simulink model "rotor_simulink"  (R2022a)
settings: Solver=VariableStepAuto  StartTime=0.1  StopTime=60  FixedStep=sample_time/10  RelTol=1e-3
values from neighbouring files (symbols this model uses):
  B_eq = rotor.B + generator.B/gearbox.ratio^2    [parameters.m]
  I_eq = rotor.I/gearbox.ratio^2 + generator.I    [main.m]    (also in parameters.m = rotor.I + generator.I/gearbox.ratio^2)
  lambda_opt = lambda_vector(lambda_pos)    [lookup_cp.m]    (also in mesh_cp.m; parameters.m = rated_values(4); reference_selection.m = 7.857)
  lambda_vector = linspace(lambda_range(1), lambda_range(2), lambda_item)    [mesh_cp.m]    (also in parameters.m)
  lookup_Pitch = zeros(3, velocity_item)    [lookup_pitch.m]    (also in lookup_pitch.mat = [0 0 0 0.5 0 0 1 0 0 1.5 0 0 ... (183 elements, 3x61)])
  omega_rated = V0_rated*lambda_opt/rotor.R    [lookup_cp.m]    (also in mesh_cp.m; parameters.m = rated_values(2); reference_selection.m = 1.008234212)
  pitch_vector = linspace(pitch_range(1), pitch_range(2), pitch_item)    [mesh_cp.m]    (also in parameters.m)
  rated_values = [11.4382324778 1.03294686619 9.86391598231 8.05263157895 0.46469860786]    [rated_values.mat]
  rho = 1.225    [main.m]    (also in parameters.m; reference_selection.m)
  sample_time = wind_speed(2,1) - wind_speed(1, 1)    [main.m]    (also in parameters.m)
  V0_rated = (rotor.P_rated/(0.5*rho*cP_max*rotor.A))^(1/3)    [lookup_cp.m]    (also in mesh_cp.m; parameters.m = rated_values(1); reference_selection.m = 11.44)
  velocity_vector = sort(velocity_vector)    [parameters.m]
  wind_speed = load('usim.dat')    [main.m]    (also in parameters.m; rotor_test.m = 25)
undefined symbols (not defined in the file or in its folder): blade, gearbox, generator, lookup_cP, omega_r, rotor
settings Model: Creator=Niccolò  LastModifiedBy=Niccolò

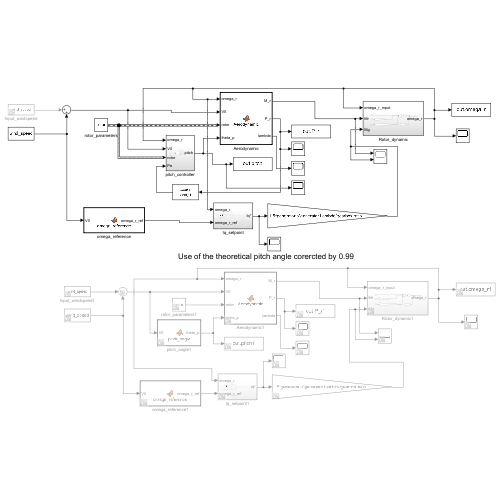
[thumbnail: Simulink's stored preview of the top-level diagram]
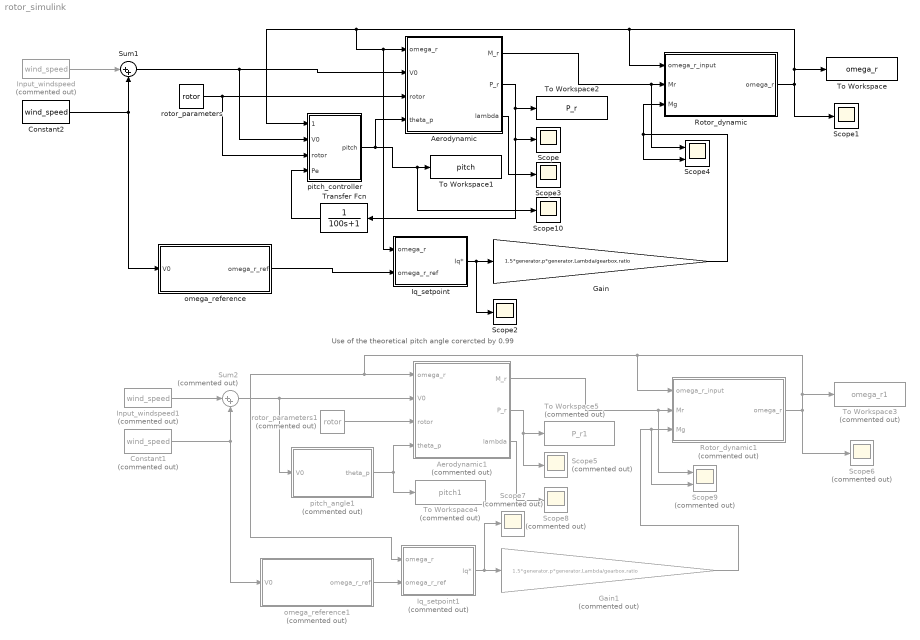
== system rotor_simulink ==
  note: Use of the theoretical pitch angle corercted by 0.99
  Aerodynamic : MATLAB Function  TreatAsAtomicUnit=on
  Aerodynamic1 : MATLAB Function  Commented=on  TreatAsAtomicUnit=on
  Constant1 : Constant  Commented=on  Value=wind_speed
  Constant2 : Constant  Value=wind_speed
  Gain : Gain  Gain=1.5*generator.p*generator.Lambda/gearbox.ratio
  Gain1 : Gain  Commented=on  Gain=1.5*generator.p*generator.Lambda/gearbox.ratio
  Input_windspeed : FromWorkspace  Commented=on  VariableName=wind_speed  SampleTime=sample_time
  Input_windspeed1 : FromWorkspace  Commented=on  VariableName=wind_speed  SampleTime=sample_time
  Iq_setpoint : Subsystem
  Iq_setpoint1 : Subsystem  Commented=on
  Rotor_dynamic : Subsystem
  Rotor_dynamic1 : Subsystem  Commented=on
  Scope{,1..3,10} (5 alike) : Scope
  Scope4 : Scope  NumInputPorts=2
  Scope{5..8} (4 alike) : Scope  Commented=on
  Scope9 : Scope  Commented=on  NumInputPorts=2
  Sum1 : Sum  Inputs=|++
  Sum2 : Sum  Commented=on  Inputs=|++
  To Workspace : ToWorkspace  VariableName=omega_r  SaveFormat=Timeseries  SampleTime=-1
  To Workspace1 : ToWorkspace  VariableName=pitch  SaveFormat=Timeseries  SampleTime=-1
  To Workspace2 : ToWorkspace  VariableName=P_r  SaveFormat=Timeseries  SampleTime=-1
  To Workspace3 : ToWorkspace  Commented=on  VariableName=omega_r1  SaveFormat=Timeseries  SampleTime=-1
  To Workspace4 : ToWorkspace  Commented=on  VariableName=pitch1  SaveFormat=Timeseries  SampleTime=-1
  To Workspace5 : ToWorkspace  Commented=on  VariableName=P_r1  SaveFormat=Timeseries  SampleTime=-1
  Transfer Fcn : TransferFcn  Denominator=[100 1]
  omega_reference : MATLAB Function  TreatAsAtomicUnit=on
  omega_reference1 : MATLAB Function  Commented=on  TreatAsAtomicUnit=on
  pitch_angle1 : MATLAB Function  Commented=on  TreatAsAtomicUnit=on
  pitch_controller : Subsystem
  rotor_parameters : Constant  Value=rotor  OutDataTypeStr=Bus: rotor_bus
  rotor_parameters1 : Constant  Commented=on  Value=rotor  OutDataTypeStr=Bus: rotor_bus
  wires:
  Input_windspeed/1 -> Sum1/1
  rotor_parameters/1 -> pitch_controller/3(rotor), Aerodynamic/3(rotor)
  Constant2/1 -> omega_reference/1(V0), Sum1/2
  omega_reference/1(omega_r_ref) -> Iq_setpoint/2(omega_r_ref)
  Iq_setpoint/1(Iq*) -> Scope2/1, Gain/1
  Gain/1 -> Rotor_dynamic/3(Mg), Scope4/2
  Aerodynamic/1(M_r) -> Scope4/1, Rotor_dynamic/2(Mr)
  Sum1/1 -> Aerodynamic/2(V0), pitch_controller/2(V0)
  Aerodynamic/3(lambda) -> Scope3/1
  Aerodynamic1/3(lambda) -> Scope8/1
  Constant1/1 -> omega_reference1/1(V0), Sum2/2
  Input_windspeed1/1 -> Sum2/1
  Sum2/1 -> Aerodynamic1/2(V0), pitch_angle1/1(V0)
  rotor_parameters1/1 -> Aerodynamic1/3(rotor)
  pitch_angle1/1(theta_p) -> Aerodynamic1/4(theta_p), To Workspace4/1
  Rotor_dynamic1/1(omega_r) -> Rotor_dynamic1/1(omega_r_input), Iq_setpoint1/1(omega_r), Aerodynamic1/1(omega_r), To Workspace3/1, Scope6/1
  omega_reference1/1(omega_r_ref) -> Iq_setpoint1/2(omega_r_ref)
  Gain1/1 -> Scope9/2, Rotor_dynamic1/3(Mg)
  Iq_setpoint1/1(Iq*) -> Scope7/1, Gain1/1
  Aerodynamic1/2(P_r) -> Scope5/1, To Workspace5/1
  Aerodynamic1/1(M_r) -> Scope9/1, Rotor_dynamic1/2(Mr)
  Aerodynamic/2(P_r) -> Transfer Fcn/1, Scope/1, To Workspace2/1
  Rotor_dynamic/1(omega_r) -> Rotor_dynamic/1(omega_r_input), pitch_controller/1(omega_r), Iq_setpoint/1(omega_r), Aerodynamic/1(omega_r), To Workspace/1, Scope1/1
  pitch_controller/1(pitch) -> Aerodynamic/4(theta_p), Scope10/1, To Workspace1/1
  Transfer Fcn/1 -> pitch_controller/4(Pe)

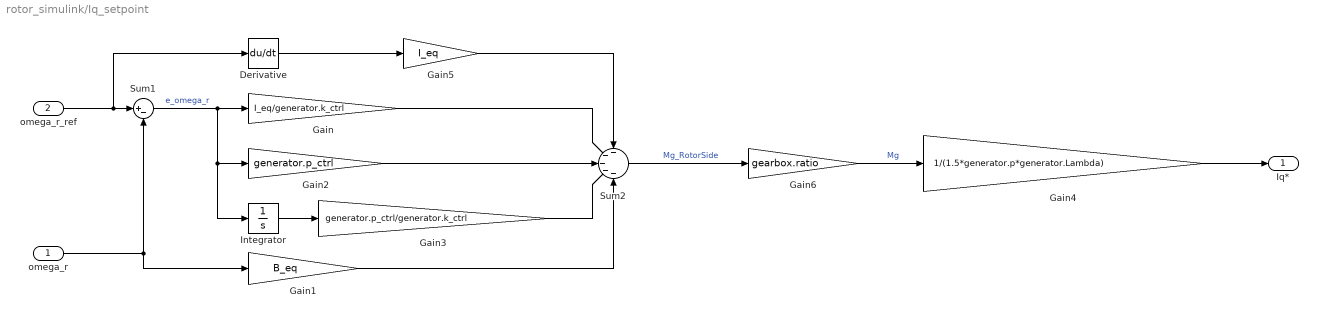
== system rotor_simulink/Iq_setpoint ==
  omega_r : Inport
  omega_r_ref : Inport  Port=2
  Derivative : Derivative
  Gain : Gain  Gain=I_eq/generator.k_ctrl
  Gain1 : Gain  Gain=B_eq
  Gain2 : Gain  Gain=generator.p_ctrl
  Gain3 : Gain  Gain=generator.p_ctrl/generator.k_ctrl
  Gain4 : Gain  Gain=1/(1.5*generator.p*generator.Lambda)
  Gain5 : Gain  Gain=I_eq
  Gain6 : Gain  Gain=gearbox.ratio
  Integrator : Integrator
  Sum1 : Sum  Inputs=|+-
  Sum2 : Sum  Inputs=-----
  Iq* : Outport
  wires:
  Gain/1 -> Sum2/2
  Sum1/1 -> Integrator/1, Gain2/1, Gain/1  "e_omega_r"
  Gain1/1 -> Sum2/5
  Gain4/1 -> Iq*/1
  omega_r_ref/1 -> Derivative/1, Sum1/1
  omega_r/1 -> Gain1/1, Sum1/2
  Integrator/1 -> Gain3/1
  Gain3/1 -> Sum2/4
  Gain2/1 -> Sum2/3
  Sum2/1 -> Gain6/1  "Mg_RotorSide"
  Gain5/1 -> Sum2/1
  Gain6/1 -> Gain4/1  "Mg"
  Derivative/1 -> Gain5/1

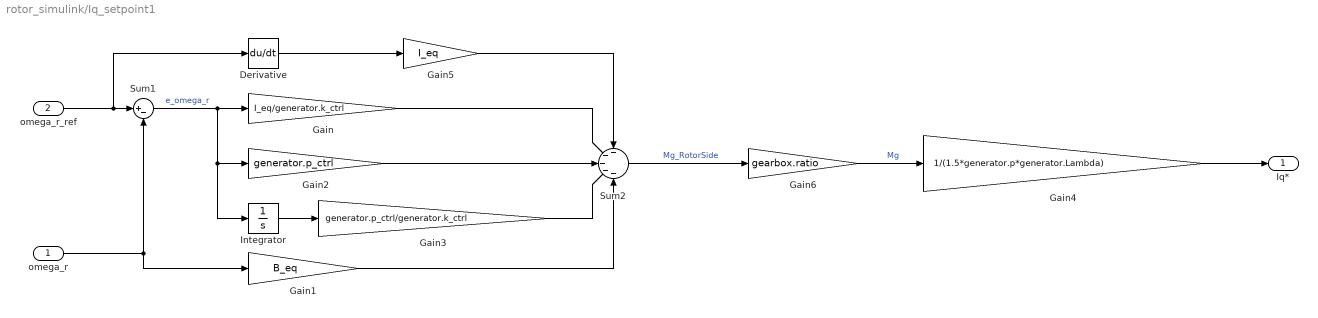
== system rotor_simulink/Iq_setpoint1 ==
  omega_r : Inport
  omega_r_ref : Inport  Port=2
  Derivative : Derivative
  Gain : Gain  Gain=I_eq/generator.k_ctrl
  Gain1 : Gain  Gain=B_eq
  Gain2 : Gain  Gain=generator.p_ctrl
  Gain3 : Gain  Gain=generator.p_ctrl/generator.k_ctrl
  Gain4 : Gain  Gain=1/(1.5*generator.p*generator.Lambda)
  Gain5 : Gain  Gain=I_eq
  Gain6 : Gain  Gain=gearbox.ratio
  Integrator : Integrator
  Sum1 : Sum  Inputs=|+-
  Sum2 : Sum  Inputs=-----
  Iq* : Outport
  wires:
  Gain/1 -> Sum2/2
  Sum1/1 -> Integrator/1, Gain2/1, Gain/1  "e_omega_r"
  Gain1/1 -> Sum2/5
  Gain4/1 -> Iq*/1
  omega_r_ref/1 -> Derivative/1, Sum1/1
  omega_r/1 -> Gain1/1, Sum1/2
  Integrator/1 -> Gain3/1
  Gain3/1 -> Sum2/4
  Gain2/1 -> Sum2/3
  Sum2/1 -> Gain6/1  "Mg_RotorSide"
  Gain5/1 -> Sum2/1
  Gain6/1 -> Gain4/1  "Mg"
  Derivative/1 -> Gain5/1

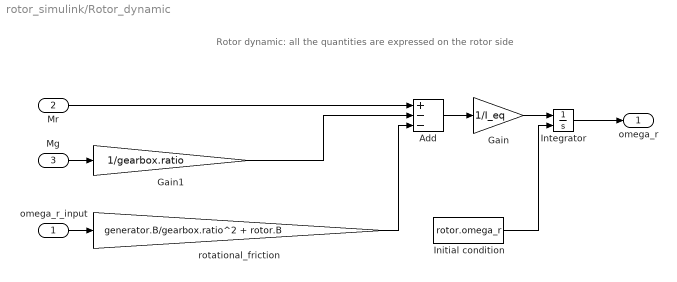
== system rotor_simulink/Rotor_dynamic ==
  note: Rotor dynamic: all the quantities are expressed on the rotor side
  omega_r_input : Inport
  Mr : Inport  Port=2
  Mg : Inport  Port=3
  Add : Sum  Inputs=+--
  Gain : Gain  Gain=1/I_eq
  Gain1 : Gain  Gain=1/gearbox.ratio
  Initial condition : Constant  Value=rotor.omega_r
  Integrator : Integrator  InitialConditionSource=external  InitialCondition=omega_r
  rotational_friction : Gain  Gain=generator.B/gearbox.ratio^2 + rotor.B
  omega_r : Outport
  wires:
  Add/1 -> Gain/1
  Gain/1 -> Integrator/1
  Mr/1 -> Add/1
  Initial condition/1 -> Integrator/2
  omega_r_input/1 -> rotational_friction/1
  rotational_friction/1 -> Add/3
  Mg/1 -> Gain1/1
  Gain1/1 -> Add/2
  Integrator/1 -> omega_r/1

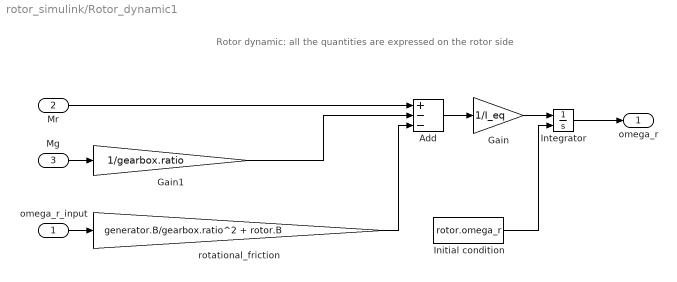
== system rotor_simulink/Rotor_dynamic1 ==
  note: Rotor dynamic: all the quantities are expressed on the rotor side
  omega_r_input : Inport
  Mr : Inport  Port=2
  Mg : Inport  Port=3
  Add : Sum  Inputs=+--
  Gain : Gain  Gain=1/I_eq
  Gain1 : Gain  Gain=1/gearbox.ratio
  Initial condition : Constant  Value=rotor.omega_r
  Integrator : Integrator  InitialConditionSource=external  InitialCondition=omega_r
  rotational_friction : Gain  Gain=generator.B/gearbox.ratio^2 + rotor.B
  omega_r : Outport
  wires:
  Add/1 -> Gain/1
  Gain/1 -> Integrator/1
  Mr/1 -> Add/1
  Initial condition/1 -> Integrator/2
  omega_r_input/1 -> rotational_friction/1
  rotational_friction/1 -> Add/3
  Mg/1 -> Gain1/1
  Gain1/1 -> Add/2
  Integrator/1 -> omega_r/1

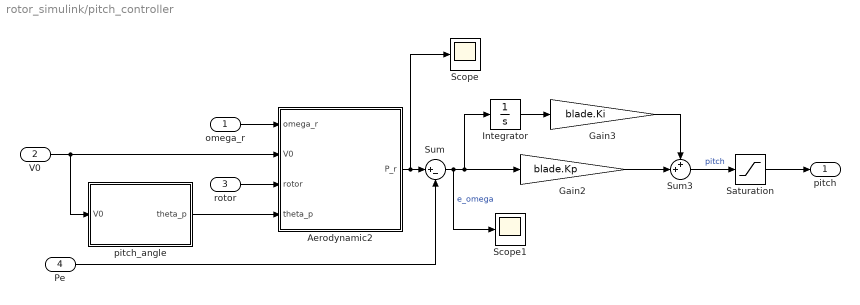
== system rotor_simulink/pitch_controller ==
  omega_r : Inport
  V0 : Inport  Port=2
  rotor : Inport  Port=3
  Pe : Inport  Port=4
  Aerodynamic2 : MATLAB Function  TreatAsAtomicUnit=on
  Gain2 : Gain  Gain=blade.Kp
  Gain3 : Gain  Gain=blade.Ki
  Integrator : Integrator
  Saturation : Saturate  UpperLimit=30*pi/180  LowerLimit=-15*pi/180
  Scope : Scope
  Scope1 : Scope
  Sum : Sum  Inputs=|+-
  Sum3 : Sum  Inputs=++|
  pitch_angle : MATLAB Function  TreatAsAtomicUnit=on
  pitch : Outport
  wires:
  Aerodynamic2/1(P_r) -> Scope/1, Sum/1
  V0/1 -> Aerodynamic2/2(V0), pitch_angle/1(V0)
  Gain3/1 -> Sum3/1
  Sum/1 -> Scope1/1, Integrator/1, Gain2/1  "e_omega"
  Gain2/1 -> Sum3/2
  Integrator/1 -> Gain3/1
  pitch_angle/1(theta_p) -> Aerodynamic2/4(theta_p)
  Pe/1 -> Sum/2
  rotor/1 -> Aerodynamic2/3(rotor)
  omega_r/1 -> Aerodynamic2/1(omega_r)
  Sum3/1 -> Saturation/1  "pitch"
  Saturation/1 -> pitch/1

== matlab function rotor_simulink/Aerodynamic1 ==
  data: omega_r input; V0 input; M_r output; P_r output; rho parameter; rotor input; theta_p input; lambda_vector parameter; pitch_vector parameter; lookup_cP parameter; lambda output
function [M_r, P_r, lambda] = Aerodynamic(omega_r, V0, rho, rotor, ...
  theta_p, lambda_vector, pitch_vector, lookup_cP) 

R = rotor.R;                  % rotor radius [m]

% retrive the cP from the look-up table
lambda = omega_r*R/V0;                                                
cP = interp2(lambda_vector, pitch_vector, lookup_cP, lambda, theta_p);

P_r = 0.5*rho*V0^3*pi*R^2*cP; % rotor power [W]
M_r = P_r/omega_r;            % rotor torque [Nm]

== matlab function rotor_simulink/pitch_controller/pitch_angle ==
  data: V0 input; theta_p output; lookup_Pitch parameter; velocity_vector parameter; rated_values parameter
function theta_p = pitch_angle(V0, lookup_Pitch, velocity_vector, ...
  rated_values)

V0_rated = rated_values(1); % rated windspeed [m/s]

if V0 < V0_rated  % below rated
  theta_p = 0;
else              % above rated
  theta_p = interp1(velocity_vector, lookup_Pitch(3, :), V0);
  theta_p = theta_p*0.99; 
end

== matlab function rotor_simulink/omega_reference1 ==
  data: V0 input; omega_r_ref output; lambda_opt parameter; rotor parameter; omega_rated parameter; V0_rated parameter
function omega_r_ref = omega_reference(V0, lambda_opt, rotor, ...
  omega_rated, V0_rated)
% This block provides the gnereator reference speed based on the expected
% rotor reference speed and the gearbox ratio

% rotor refernce speed
if V0 < V0_rated    % below rated -> MPPT
  omega_r_ref = lambda_opt*V0/rotor.R;
else                % above rated -> power limitation
  omega_r_ref = omega_rated;
end

== matlab function rotor_simulink/Aerodynamic ==
  data: omega_r input; V0 input; M_r output; P_r output; rho parameter; rotor input; theta_p input; lambda_vector parameter; pitch_vector parameter; lookup_cP parameter; lambda output
function [M_r, P_r, lambda] = Aerodynamic(omega_r, V0, rho, rotor, ...
  theta_p, lambda_vector, pitch_vector, lookup_cP) 

R = rotor.R;                  % rotor radius [m]

% retrive the cP from the look-up table
lambda = omega_r*R/V0;                                                
cP = interp2(lambda_vector, pitch_vector, lookup_cP, lambda, theta_p);

P_r = 0.5*rho*V0^3*pi*R^2*cP; % rotor power [W]
M_r = P_r/omega_r;            % rotor torque [Nm]

== matlab function rotor_simulink/omega_reference ==
  data: V0 input; omega_r_ref output; lambda_opt parameter; rotor parameter; omega_rated parameter; V0_rated parameter
function omega_r_ref = omega_reference(V0, lambda_opt, rotor, ...
  omega_rated, V0_rated)
% This block provides the gnereator reference speed based on the expected
% rotor reference speed and the gearbox ratio

% rotor refernce speed
if V0 < V0_rated    % below rated -> MPPT
  omega_r_ref = lambda_opt*V0/rotor.R;
else                % above rated -> power limitation
  omega_r_ref = omega_rated;
end

== matlab function rotor_simulink/pitch_angle1 ==
  data: V0 input; theta_p output; lookup_Pitch parameter; velocity_vector parameter; rated_values parameter
function theta_p = pitch_angle(V0, lookup_Pitch, velocity_vector, ...
  rated_values)

V0_rated = rated_values(1); % rated windspeed [m/s]

if V0 < V0_rated  % below rated
  theta_p = 0;
else              % above rated
  theta_p = interp1(velocity_vector, lookup_Pitch(3, :), V0);
  theta_p = theta_p*0.99; 
end

== matlab function rotor_simulink/pitch_controller/Aerodynamic2 ==
  data: omega_r input; V0 input; P_r output; rho parameter; rotor input; theta_p input; lambda_vector parameter; pitch_vector parameter; lookup_cP parameter
function P_r  = Aerodynamic(omega_r, V0, rho, rotor, ...
  theta_p, lambda_vector, pitch_vector, lookup_cP) 

R = rotor.R;                  % rotor radius [m]

% retrive the cP from the look-up table
lambda = omega_r*R/V0;                                                
cP = interp2(lambda_vector, pitch_vector, lookup_cP, lambda, theta_p);

P_r = 0.5*rho*V0^3*pi*R^2*cP; % rotor power [W]
